simulink model "Exercise121"  (R2017a)
settings: Solver=VariableStepAuto  StartTime=0.0  StopTime=10.0  MaxStep=0.002  RelTol=1e-3
undefined symbols (not defined in the file): Fin_Val, Step_Time, Ts
settings Model: Creator=JakobLab  LastModifiedBy=JakobLab

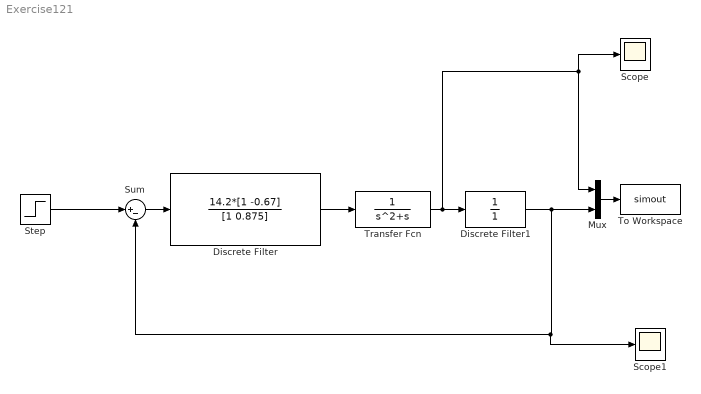
== system Exercise121 ==
  Discrete Filter : DiscreteFilter  Numerator=14.2*[1 -0.67]  Denominator=[1 0.875]  SampleTime=Ts
  Discrete Filter1 : DiscreteFilter  Numerator=1  Denominator=1  SampleTime=Ts
  Mux : Mux  Inputs=2
  Scope : Scope
  Scope1 : Scope
  Step : Step  Time=Step_Time  After=Fin_Val  SampleTime=0
  Sum : Sum  Inputs=|+-
  To Workspace : ToWorkspace  VariableName=simout  SaveFormat=Structure With Time  SampleTime=-1
  Transfer Fcn : TransferFcn  Denominator=[1 1 0]
  wires:
  Step/1 -> Sum/1
  Sum/1 -> Discrete Filter/1
  Discrete Filter/1 -> Transfer Fcn/1
  Transfer Fcn/1 -> Scope/1, Mux/1, Discrete Filter1/1
  Mux/1 -> To Workspace/1
  Discrete Filter1/1 -> Mux/2, Scope1/1, Sum/2
